simulink model "feedback_harness"  (R2019b)
settings: Solver=ode4  StartTime=0.0  StopTime=ToA(end)  FixedStep=0.001  RelTol=1e-3
model workspace (MAT data in the model file):
  traj = waypointTrajectory
  traj.any.ClassNameForLoadTimeEval = 'waypointTrajectory'
  traj.any.MajorVersionNumber = 9
  traj.any.MinorVersionNumber = 1792
  traj.any.ChildClassData.SampleRate = 100
  traj.any.ChildClassData.SamplesPerFrame = 1
  traj.any.ChildClassData.Waypoints = [0  0  0; 0  1  0; 1  1  0; 1  0  0; 0  0  0]
  traj.any.ChildClassData.TimeOfArrival = [0; 1; 2; 3; 4]
  traj.any.ChildClassData.Velocities = []
  traj.any.ChildClassData.RotMats = reshape([1 0 0 0 1 0 0 0 1 0.707106781187 -0.707106781187 0 0.707106781187 0.707106781187 0 0 0 1 -0.707106781187 -0.707106781187 0 0.707106781187 -0.707106781187 0 0 0 1 -0.707106781187 0.707106781187 0 -0.707106781187 -0.707106781187 0 0 0 1 1 0 0 0 1 0 0 0 1], [3 3 5])
  traj.any.ChildClassData.Quaternions = quaternion
  traj.any.ChildClassData.Quaternions.a = [1; 0.923879532511; 0.382683432365; -0.382683432365; 1]
  traj.any.ChildClassData.Quaternions.b = [0; 0; 0; 0; 0]
  traj.any.ChildClassData.Quaternions.c = [0; 0; 0; 0; 0]
  traj.any.ChildClassData.Quaternions.d = [0; 0.382683432365; 0.923879532511; 0.923879532511; 0]
  traj.any.ChildClassData.IsWaypointsSpecified = 1
  traj.any.ChildClassData.IsTimeOfArrivalSpecified = 1
  traj.any.ChildClassData.IsVelocitiesSpecified = 0
  traj.any.ChildClassData.IsOrientationSpecified = 1
  traj.any.ChildClassData.IsOrientationQuaternion = 1
  traj.any.ChildClassData.CurrentPoseValidStatus = 0
  traj.any.SuperClassData = []
undefined symbols (not defined in the file): pos_ref, psi_ref, psidot_ref, t_ref, vel_ref
libraries: vrlib x5, aerolibfltsims x3, simulink x2, sldrtlib x1
settings Model: ModifiedByFormat=The MathWorks Inc.  NumberOfSteps=100  SnapshotBufferSize=3  SnapshotInterval=100  ExtModeTrigDuration=10  OrderedModelArguments=off  Creator=The MathWorks, Inc.  LastModifiedBy=The MathWorks Inc.
settings DataIOCC: LimitDataPoints=on  SaveFormat=Array  SaveOutput=off  SaveTime=off  ReturnWorkspaceOutputs=off
settings OptimizationCC: ExpressionDepthLimit=2147483647  LifeSpan=1
settings DebuggingCC: UnderspecifiedInitializationDetection=Classic  MergeDetectMultiDrivingBlocksExec=none  SolverPrmCheckMsg=warning  FcnCallInpInsideContextMsg=warning  StateNameClashWarn=warning  SFUnexpectedBacktrackingDiag=warning  SFNoUnconditionalDefaultTransitionDiag=warning  SFExecutionAtInitializationDiag=none  ArithmeticOperatorsInVariantConditions=warning
settings HardwareCC: ProdBitPerPointer=32  ProdBitPerSizeT=32  ProdBitPerPtrDiffT=32  ProdLargestAtomicFloat=None  ProdIntDivRoundTo=Undefined  ProdEndianess=Unspecified  ProdWordSize=32  ProdHWDeviceType=32-bit Generic
settings ModelReferenceCC: PropagateSignalLabelsOutOfModel=off
settings SFSimCC: SimUseLocalCustomCode=off  CustomCodeUndefinedFunction=UseInterfaceOnly
settings RTWCC: RTWUseLocalCustomCode=off
settings CodeAppCC: StateflowObjectComments=on
settings GRTTargetCC: TargetLangStandard=C89/C90 (ANSI)  GeneratePreprocessorConditionals=Disable all  CombineOutputUpdateFcns=off  GRTInterface=on
settings ConfigComp: CovMetricSettings=dw  CovHtmlReporting=on  CovSaveCumulativeToWorkspaceVar=on  CovSaveSingleToWorkspaceVar=on  CovExternalEMLEnable=off  CovSFcnEnable=off

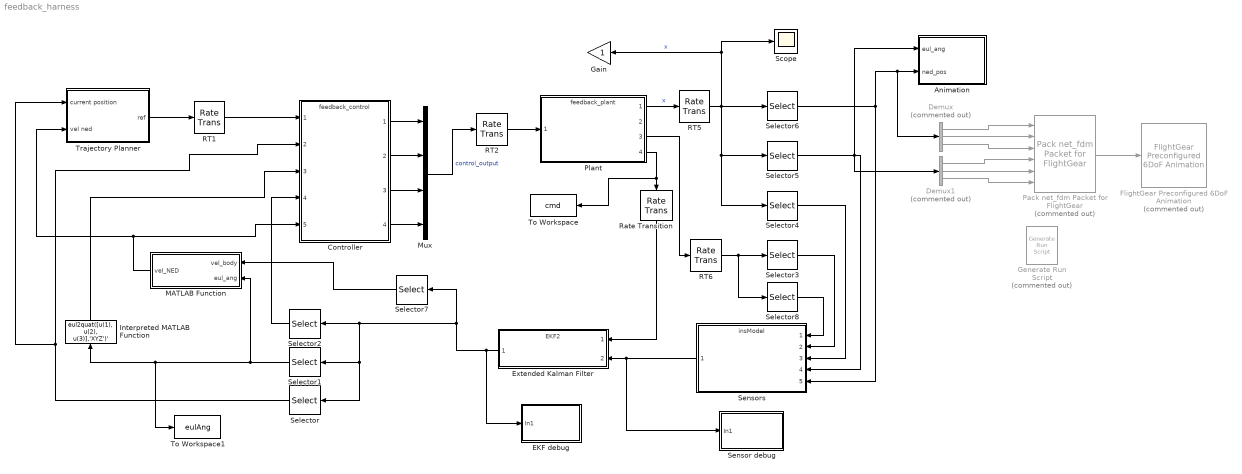
== system feedback_harness ==
  Animation : Subsystem
  Controller : ModelReference  ModelNameDialog=feedback_control.slx  SimulationMode=Normal  ModelReferenceVersion=1.124
  Demux : Demux  Commented=on  Outputs=3
  Demux1 : Demux  Commented=on  Outputs=3
  EKF debug : Subsystem
  Extended Kalman Filter : ModelReference  ModelNameDialog=EKF2  SimulationMode=Normal  ModelReferenceVersion=1.76
  FlightGear Preconfigured 6DoF Animation : aerolibfltsims/FlightGear Preconfigured 6DoF Animation  Commented=on  xFlightGearVersion=v2018.2  DestinationIpAddress=127.0.0.1  DestinationPort=5502  SampleTime=0.1  packetVersion=24
      settings: SourceProductName=Aerospace Blockset
  Gain : Gain
  Generate Run Script : aerolibfltsims/Generate Run Script  Commented=on  Architecture=Default  dataFlow=Send  GeometryModelName=HL20  AirportId=KSFO  RunwayId=10L  InitialAltitude=7224  InitialHeading=113  OffsetDistance=4.72  OffsetAzimuth=0  InstallScenery=off  DisableShaders=off  OriginAddress=127.0.0.1  DestinationPort=5502  OriginPort=5505  LocalAddress=127.0.0.1  OutputFileName=runfg.bat  FlightGearBaseDirectory=C:\Program Files\FlightGear
  Interpreted MATLAB Function : MATLABFcn  MATLABFcn=eul2quat([u(1), u(2), u(3)],'XYZ')'  OutputDimensions=4
  MATLAB Function : MATLAB Function  TreatAsAtomicUnit=on
  Mux : Mux
  Pack net_fdm Packet for FlightGear : aerolibfltsims/Pack net_fdm Packet for FlightGear  Commented=on  FlightGearVersion=v2018.2  ShowPositionAttitudeInputs=on  ShowVelocityAccelerationInputs=off  ShowControlSurfacePositionInputs=off  ShowEngineFuelInputs=off  ShowLandingGearInputs=off  ShowEnvironmentInputs=off  SampleTime=0.1  packetVersion=24
      settings: SourceProductName=Aerospace Blockset  SourceProductBaseCode=AE
  Plant : ModelReference  ModelNameDialog=feedback_plant.slx  SimulationMode=Normal  ModelReferenceVersion=1.93
  RT1 : RateTransition  OutPortSampleTimeOpt=Inherit  OutPortSampleTime=0.01
  RT2 : RateTransition  OutPortSampleTimeOpt=Inherit  OutPortSampleTime=0.001
  RT5 : RateTransition  OutPortSampleTimeOpt=Inherit  OutPortSampleTime=0.01
  RT6 : RateTransition  OutPortSampleTimeOpt=Inherit  OutPortSampleTime=0.01
  Rate Transition : RateTransition
  Scope : Scope
  Selector : Selector  InputPortWidth=12  IndexOptions=Index vector (dialog)  Indices=[1:3]  OutputSizes=1
  Selector1 : Selector  InputPortWidth=12  IndexOptions=Index vector (dialog)  Indices=[4:6]  OutputSizes=1
  Selector2 : Selector  InputPortWidth=12  IndexOptions=Index vector (dialog)  Indices=[10:12]  OutputSizes=1
  Selector3 : Selector  InputPortWidth=12  IndexOptions=Index vector (dialog)  Indices=[7:9]  OutputSizes=1
  Selector4 : Selector  InputPortWidth=12  IndexOptions=Index vector (dialog)  Indices=[10:12]  OutputSizes=1
  Selector5 : Selector  InputPortWidth=12  IndexOptions=Index vector (dialog)  Indices=[4:6]  OutputSizes=1
  Selector6 : Selector  InputPortWidth=12  IndexOptions=Index vector (dialog)  Indices=[1:3]  OutputSizes=1
  Selector7 : Selector  InputPortWidth=12  IndexOptions=Index vector (dialog)  Indices=[7:9]  OutputSizes=1
  Selector8 : Selector  InputPortWidth=12  IndexOptions=Index vector (dialog)  Indices=[1:3]  OutputSizes=1
  Sensor debug : Subsystem
  Sensors : ModelReference  ModelNameDialog=insModel  SimulationMode=Normal  ModelReferenceVersion=1.43
  To Workspace : ToWorkspace  VariableName=cmd  SaveFormat=Timeseries  SampleTime=-1
  To Workspace1 : ToWorkspace  VariableName=eulAng  SaveFormat=Timeseries  SampleTime=-1
  Trajectory Planner : Subsystem
  wires:
  Mux/1 -> RT2/1  "control_output"
  RT5/1 -> Gain/1, Scope/1, Selector4/1, Selector5/1, Selector6/1  "x"
  RT1/1 -> Controller/1
  RT2/1 -> Plant/1
  Controller/1 -> Mux/1
  Controller/2 -> Mux/2
  Controller/3 -> Mux/3
  Controller/4 -> Mux/4
  Selector/1 -> Controller/2, Trajectory Planner/1(current position)
  Interpreted MATLAB Function/1 -> Controller/3
  MATLAB Function/1(vel_NED) -> Trajectory Planner/2(vel ned), Controller/5
  Selector2/1 -> Controller/4
  Trajectory Planner/1(ref) -> RT1/1
  Selector1/1 -> MATLAB Function/2(eul_ang), To Workspace1/1, Interpreted MATLAB Function/1
  Sensors/1 -> Extended Kalman Filter/2, Sensor debug/1(In1)
  Plant/3 -> RT6/1
  Selector3/1 -> Sensors/2
  Selector4/1 -> Sensors/3
  Selector5/1 -> Demux1/1, Animation/1(eul_ang), Sensors/4
  Selector6/1 -> Demux/1, Animation/2(ned_pos), Sensors/5
  RT6/1 -> Selector8/1, Selector3/1
  Selector7/1 -> MATLAB Function/1(vel_body)
  Plant/4 -> To Workspace/1, Rate Transition/1
  Rate Transition/1 -> Extended Kalman Filter/1
  Plant/1 -> RT5/1  "x"
  Extended Kalman Filter/1 -> Selector7/1, Selector/1, Selector1/1, Selector2/1, EKF debug/1(In1)
  Selector8/1 -> Sensors/1
  Pack net_fdm Packet for FlightGear/1 -> FlightGear Preconfigured 6DoF Animation/1
  Demux/2 -> Pack net_fdm Packet for FlightGear/2
  Demux/1 -> Pack net_fdm Packet for FlightGear/1
  Demux/3 -> Pack net_fdm Packet for FlightGear/3
  Demux1/2 -> Pack net_fdm Packet for FlightGear/5
  Demux1/1 -> Pack net_fdm Packet for FlightGear/4
  Demux1/3 -> Pack net_fdm Packet for FlightGear/6

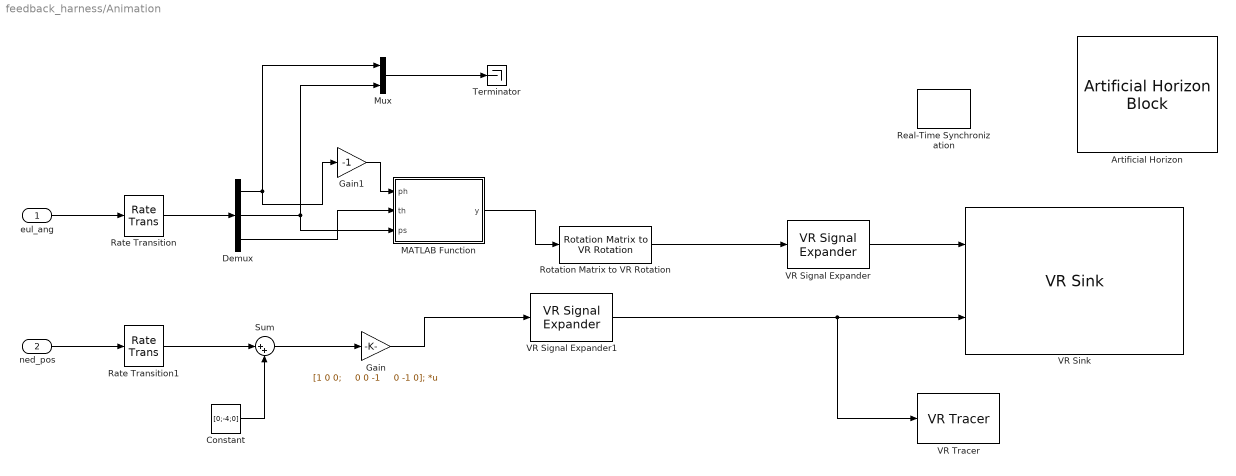
== system feedback_harness/Animation ==
  eul_ang : Inport
  ned_pos : Inport  Port=2
  Artificial Horizon : ArtificialHorizonBlock
  Constant : Constant  Value=[0;-4;0]
  Demux : Demux  Outputs=3
  Gain : Gain  Gain=|  Multiplication=Matrix(K*u)
      | [1 0 0;
      |     0 0 -1
      |     0 -1 0];
  Gain1 : Gain  Gain=-1
  MATLAB Function : MATLAB Function  TreatAsAtomicUnit=on
  Mux : Mux  Inputs=2
  Rate Transition : RateTransition  OutPortSampleTime=0.1
  Rate Transition1 : RateTransition  OutPortSampleTime=0.1
  Real-Time Synchronization : sldrtlib/Real-Time Synchronization  SampleTime=0.1  MaxMissedTicks=10  ShowMissedTicks=off  YieldWhenWaiting=off
  Rotation Matrix to VR Rotation : vrlib/Utilities/Rotation Matrix to VR Rotation  maxzero=1e-12
      settings: SourceProductName=Simulink  SourceProductBaseCode=SL
  Sum : Sum  Inputs=|++
  Terminator : Terminator
  VR Signal Expander : vrlib/VR Signal Expander  outwidth=4  outidx=[1:4]
      settings: SourceProductName=Simulink
  VR Signal Expander1 : vrlib/VR Signal Expander  outwidth=3  outidx=[1:3]
      settings: SourceProductName=Simulink
  VR Sink : vrlib/VR Sink  InstantiateOnLoad=on  SampleTime=0.1  ViewEnable=on  RemoteChange=off  RemoteView=off  FieldsWritten=UAV.rotation.4.1.1.double#UAV.translation.3.1.1.double  WorldFileName=C:\Users\david\OneDrive - Politecnico di Torino\Tesi droni\Simulink Projects\SMC\animation\uav_scene.x3dv  WorldDescription=UAV Competition Scene  AutoView=off  VideoDimensions=[]  AllowVariableSize=off
      settings: SourceProductName=Simulink
  VR Tracer : vrlib/VR Tracer  VrmlFile=C:\Users\david\OneDrive - Politecnico di Torino\Tesi droni\Simulink Projects\SMC\animation\uav_scene.x3dv  MarkerName=Sphere  UseLines=on  UseTriads=on  MarkerScale=[0.1 0.1 0.1]  MarkerColorSelection=Selected from color list  MarkerColor=red  rgbval=[1 0 0]  Ts=0.5  ForceViewerOpen=off  ConnectPlane=off  PlaneCoeff=[0 1 0 0]  ConnectPoint=None  PointCoord=[0 0 0]
      settings: SourceProductName=Simulink  SourceProductBaseCode=SL
  wires:
  ned_pos/1 -> Rate Transition1/1
  eul_ang/1 -> Rate Transition/1
  Demux/1 -> Gain1/1, Mux/1
  Rotation Matrix to VR Rotation/1 -> VR Signal Expander/1
  Rate Transition1/1 -> Sum/1
  Rate Transition/1 -> Demux/1
  Mux/1 -> Terminator/1
  VR Signal Expander/1 -> VR Sink/1
  VR Signal Expander1/1 -> VR Tracer/1, VR Sink/2
  Gain/1 -> VR Signal Expander1/1
  MATLAB Function/1(y) -> Rotation Matrix to VR Rotation/1
  Demux/3 -> MATLAB Function/2(th)
  Demux/2 -> MATLAB Function/3(ps), Mux/2
  Gain1/1 -> MATLAB Function/1(ph)
  Sum/1 -> Gain/1
  Constant/1 -> Sum/2

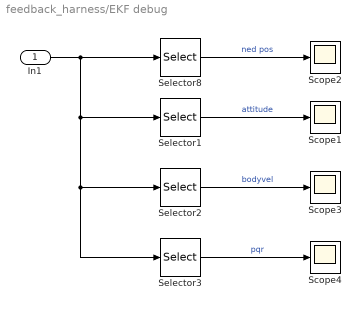
== system feedback_harness/EKF debug ==
  In1 : Inport
  Scope{1..4} (4 alike) : Scope
  Selector1 : Selector  InputPortWidth=12  IndexOptions=Index vector (dialog)  Indices=[4:6]  OutputSizes=1
  Selector2 : Selector  InputPortWidth=12  IndexOptions=Index vector (dialog)  Indices=[7:9]  OutputSizes=1
  Selector3 : Selector  InputPortWidth=12  IndexOptions=Index vector (dialog)  Indices=[10:12]  OutputSizes=1
  Selector8 : Selector  InputPortWidth=12  IndexOptions=Index vector (dialog)  Indices=[1:3]  OutputSizes=1
  wires:
  Selector8/1 -> Scope2/1  "ned pos"
  Selector1/1 -> Scope1/1  "attitude"
  Selector2/1 -> Scope3/1  "bodyvel"
  Selector3/1 -> Scope4/1  "pqr"
  In1/1 -> Selector3/1, Selector2/1, Selector1/1, Selector8/1

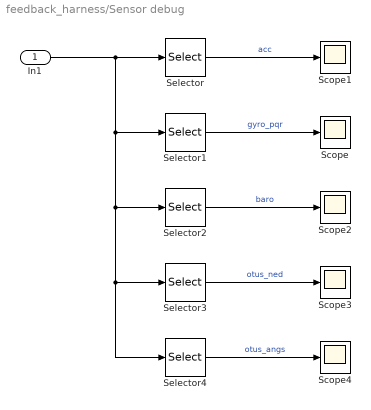
== system feedback_harness/Sensor debug ==
  In1 : Inport
  Scope{,1..4} (5 alike) : Scope
  Selector : Selector  InputPortWidth=13  IndexOptions=Index vector (dialog)  Indices=[1:3]  OutputSizes=1
  Selector1 : Selector  InputPortWidth=13  IndexOptions=Index vector (dialog)  Indices=[4:6]  OutputSizes=1
  Selector2 : Selector  InputPortWidth=13  IndexOptions=Index vector (dialog)  Indices=7  OutputSizes=1
  Selector3 : Selector  InputPortWidth=13  IndexOptions=Index vector (dialog)  Indices=[8:10]  OutputSizes=1
  Selector4 : Selector  InputPortWidth=13  IndexOptions=Index vector (dialog)  Indices=[11:13]  OutputSizes=1
  wires:
  In1/1 -> Selector4/1, Selector3/1, Selector2/1, Selector1/1, Selector/1
  Selector/1 -> Scope1/1  "acc"
  Selector1/1 -> Scope/1  "gyro_pqr"
  Selector2/1 -> Scope2/1  "baro"
  Selector3/1 -> Scope3/1  "otus_ned"
  Selector4/1 -> Scope4/1  "otus_angs"

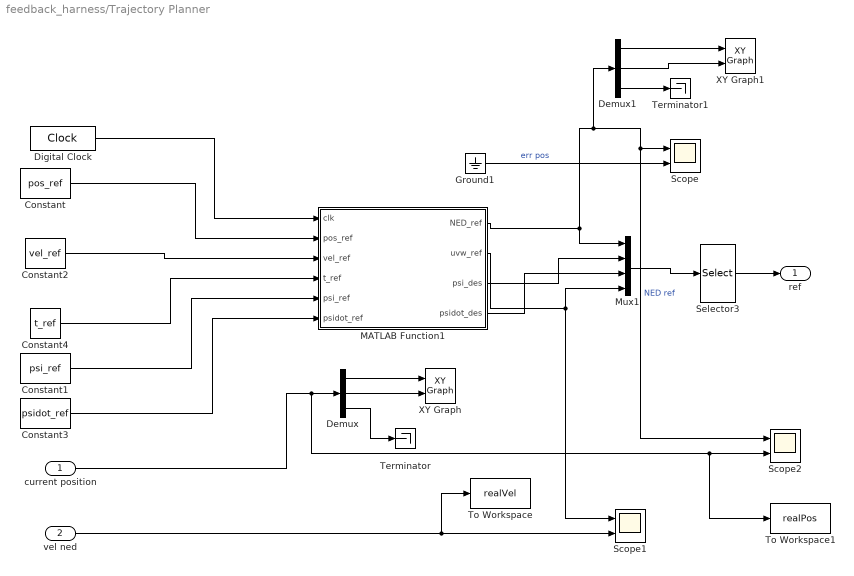
== system feedback_harness/Trajectory Planner ==
  current position : Inport
  vel ned : Inport  Port=2
  Constant : Constant  Value=pos_ref
  Constant1 : Constant  Value=psi_ref
  Constant2 : Constant  Value=vel_ref
  Constant3 : Constant  Value=psidot_ref
  Constant4 : Constant  Value=t_ref
  Demux : Demux  Outputs=3
  Demux1 : Demux  Outputs=3
  Digital Clock : DigitalClock  SampleTime=-1
  Ground1 : Ground
  MATLAB Function1 : MATLAB Function  TreatAsAtomicUnit=on
  Mux1 : Mux
  Scope : Scope  NumInputPorts=2
  Scope1 : Scope  NumInputPorts=2
  Scope2 : Scope  NumInputPorts=2
  Selector3 : Selector  InputPortWidth=9  IndexOptions=Index vector (dialog)  Indices=[1 7 2 8 4 5 3 9]  OutputSizes=1
  Terminator : Terminator
  Terminator1 : Terminator
  To Workspace : ToWorkspace  VariableName=realVel  SaveFormat=Timeseries  SampleTime=-1
  To Workspace1 : ToWorkspace  VariableName=realPos  SaveFormat=Timeseries  SampleTime=-1
  XY Graph : simulink/Sinks/XY Graph  xmin=-20  xmax=20  ymin=-20  ymax=20  st=-1
  XY Graph1 : simulink/Sinks/XY Graph  xmin=-20  xmax=20  ymin=-20  ymax=20  st=-1
  ref : Outport  VectorParamsAs1DForOutWhenUnconnected=off
  wires:
  MATLAB Function1/2(uvw_ref) -> Mux1/4, Scope1/1
  MATLAB Function1/3(psi_des) -> Mux1/2
  Mux1/1 -> Selector3/1
  MATLAB Function1/1(NED_ref) -> Mux1/1, Demux1/1, Scope2/1, Scope/1  "NED ref"
  Selector3/1 -> ref/1
  Constant/1 -> MATLAB Function1/2(pos_ref)
  Constant2/1 -> MATLAB Function1/3(vel_ref)
  current position/1 -> To Workspace1/1, Scope2/2, Demux/1
  Ground1/1 -> Scope/2  "err pos"
  Demux/2 -> XY Graph/2
  Demux/1 -> XY Graph/1
  Demux/3 -> Terminator/1
  Demux1/1 -> XY Graph1/1
  Demux1/2 -> XY Graph1/2
  Demux1/3 -> Terminator1/1
  vel ned/1 -> To Workspace/1, Scope1/2
  Constant4/1 -> MATLAB Function1/4(t_ref)
  Digital Clock/1 -> MATLAB Function1/1(clk)
  Constant1/1 -> MATLAB Function1/5(psi_ref)
  Constant3/1 -> MATLAB Function1/6(psidot_ref)
  MATLAB Function1/4(psidot_des) -> Mux1/3

== matlab function feedback_harness/MATLAB Function ==
  data: vel_body input; vel_NED output; eul_ang input
function vel_NED = body2NED(vel_body,eul_ang)

ph = eul_ang(1);
th = eul_ang(2);
ps = eul_ang(3);

Rb_ned = [ cos(th)*cos(ps), cos(th)*sin(ps), -sin(th)
            -cos(ph)*sin(ps) + sin(ph)*sin(th)*cos(ps), cos(ph)...
                *cos(ps) + sin(ph)*sin(th)*sin(ps), sin(ph)*cos(th)
            sin(ph)*sin(ps) + cos(ph)*sin(th)*cos(ps), -sin(ph)...
            *cos(ps) + cos(ph)*sin(th)*sin(ps), cos(ph)*cos(th) ];
        
vel_NED = Rb_ned'*vel_body;

end

== matlab function feedback_harness/Animation/MATLAB Function ==
  data: ph input; y output; th input; ps input
function y = fcn(ph,th,ps)

Rb_ned = [ cos(th)*cos(ps), cos(th)*sin(ps), -sin(th)
            -cos(ph)*sin(ps) + sin(ph)*sin(th)*cos(ps), cos(ph)...
                *cos(ps) + sin(ph)*sin(th)*sin(ps), sin(ph)*cos(th)
            sin(ph)*sin(ps) + cos(ph)*sin(th)*cos(ps), -sin(ph)...
            *cos(ps) + cos(ph)*sin(th)*sin(ps), cos(ph)*cos(th) ];
Rx = [1 0 0;
    0 1 0
    0 0 1];
        
y = Rx*Rb_ned';

== matlab function feedback_harness/Trajectory Planner/MATLAB Function1 ==
  data: clk input; NED_ref output; uvw_ref output; psi_des output; pos_ref input; vel_ref input; t_ref input; psi_ref input; psidot_ref input; psidot_des output
function [ NED_ref, uvw_ref, psi_des, psidot_des]  = trajectoryPlanner(clk,pos_ref,vel_ref,t_ref, psi_ref, psidot_ref)

currTime = find(clk >= t_ref);
NED_ref = pos_ref(currTime(end),:);
uvw_ref = vel_ref(currTime(end),:);
psi_des = psi_ref(currTime(end),:);
psidot_des = psidot_ref(currTime(end),:);
end
